simulink library "aeroblk_lib_wf_3dof"  (Simulink 6.0)
settings: Solver=ode45  SolverMode=SingleTasking  StartTime=0.0  StopTime=10.0  RelTol=1e-3
values from neighbouring files (symbols this model uses):
  wf_alphaa = 4.12    [aeroblk_wf_3dof_data.m]
  wf_B3 = 0.06    [aeroblk_wf_3dof_data.m]
  wf_c = 6.5    [aeroblk_wf_3dof_data.m]
  wf_cg = 29    [aeroblk_wf_3dof_data.m]
  wf_cp_e = 112    [aeroblk_wf_3dof_data.m]
  wf_gravity = 32.17    [aeroblk_wf_3dof_data.m]
  wf_H = 16.9    [aeroblk_wf_3dof_data.m]
  wf_incidence = 8    [aeroblk_wf_3dof_data.m]
  wf_Q2 = 1.8    [aeroblk_wf_3dof_data.m]
  wf_Q4 = 2.0    (= 2)    [aeroblk_wf_3dof_data.m]
  wf_sref = 510    [aeroblk_wf_3dof_data.m]
  wf_w2e = 9.7    [aeroblk_wf_3dof_data.m]
  wf_weight = 750    [aeroblk_wf_3dof_data.m]
  wf_z1 = 15    [aeroblk_wf_3dof_data.m]
  wf_z2 = 23    [aeroblk_wf_3dof_data.m]
  wf_z3 = 13    [aeroblk_wf_3dof_data.m]
libraries: simulink x23, aerolibconvert x10, aerolibasang x2, aerolib3dof2 x1, aerolibutil x1, aerolibtransform2 x1, aerolibatmos2 x1, aerolibwind2 x1, aerolibgravity2 x1
settings Model: Creator=The MathWorks Inc.  LastModifiedBy=batserve  ExtModeAutoUpdateStatusClock=off
settings OptimizationCC: BooleanDataType=off
settings DebuggingCC: CheckExecutionContextPreStartOutputMsg=on  CheckExecutionContextRuntimeOutputMsg=on  SolverPrmCheckMsg=none
settings HardwareCC: TargetUnknown=on

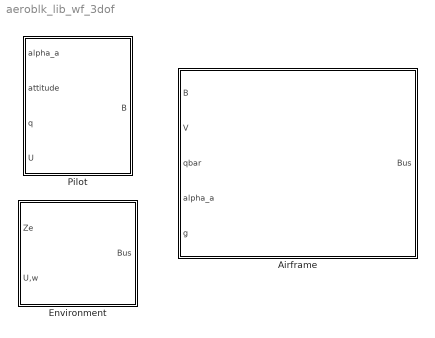
== system aeroblk_lib_wf_3dof ==
  Airframe : Subsystem  PropExecContextAcrossSSBoundary=on
      mask Display: image(imread('aeroblk_wf.jpg'))
  Environment : Subsystem  PropExecContextAcrossSSBoundary=on
      mask Display: image(imread('aeroblk_wf_atmos.jpg'))
  Pilot : Subsystem  PropExecContextAcrossSSBoundary=on
      mask Display: image(imread('aeroblk_orville.jpg'))

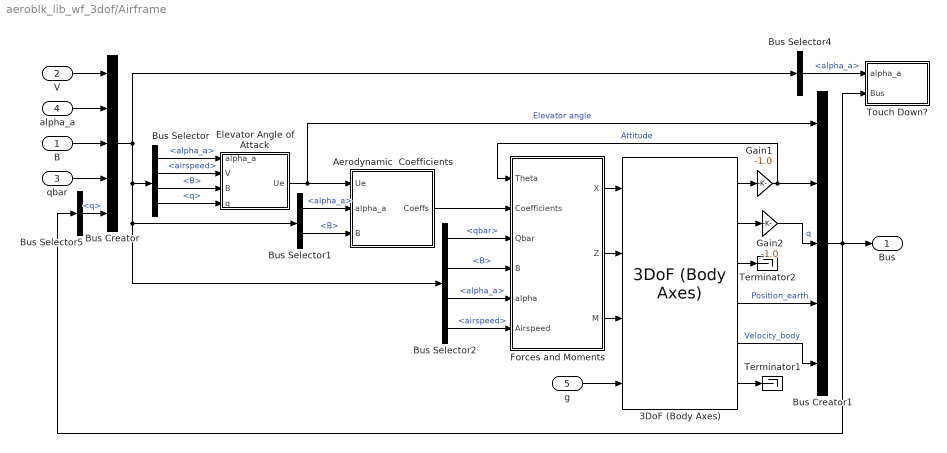
== system aeroblk_lib_wf_3dof/Airframe ==
  "B " : Inport  Port=1  LatchInput=off
  V : Inport  Port=2  LatchInput=off
  qbar : Inport  Port=3  LatchInput=off
  alpha_a : Inport  Port=4  LatchInput=off
  g : Inport  Port=5  LatchInput=off
  3DoF (Body Axes) : aerolib3dof2/3DoF (Body Axes)  units=English (Velocity in ft/s)  mtype=Fixed  v_ini=47.26  theta_ini=-(wf_alphaa-wf_incidence)*pi/180  alpha_ini=wf_alphaa*pi/180  q_ini=wf_q  pos_ini=[0 -0.1]  mass=wf_weight/wf_gravity  mass_e=0.5  mass_f=3.0  Iyy=wf_inertia  Iyy_e=0.5  Iyy_f=3.0  g_in=External  g=wf_gravity
  Aerodynamic  Coefficients : Subsystem  PropExecContextAcrossSSBoundary=on
  Bus Creator : BusCreator  DialogController=Simulink.DDGSource_Bus  Inputs=5
  Bus Creator1 : BusCreator  DialogController=Simulink.DDGSource_Bus  Inputs=5
  Bus Selector : BusSelector  DialogController=Simulink.DDGSource_Bus  OutputSignals=alpha_a,airspeed,B,q
  Bus Selector1 : BusSelector  DialogController=Simulink.DDGSource_Bus  OutputSignals=alpha_a,B
  Bus Selector2 : BusSelector  DialogController=Simulink.DDGSource_Bus  OutputSignals=qbar,B,alpha_a,airspeed
  Bus Selector4 : BusSelector  DialogController=Simulink.DDGSource_Bus  OutputSignals=alpha_a
  Bus Selector5 : BusSelector  DialogController=Simulink.DDGSource_Bus  OutputSignals=q
  "Elevator Angle of Attack " : Subsystem  PropExecContextAcrossSSBoundary=on
  Forces and Moments : Subsystem  PropExecContextAcrossSSBoundary=on
      mask Display:
      | port_label('input',1,'\theta','texmode','on');
      | port_label('input',2,'Coeffs','texmode','on');
      | port_label('input',3,'q_{bar}','texmode','on');
      | port_label('input',4,'B','texmode','on');
      | port_label('input',5,'\alpha','texmode','on');
      | port_label('input',6,'Airspeed','texmode','on');
      | port_label('output',1,'F_x','texmode','on');
      | port_label('output',2,'F_z','texmode','on');
      | port_label('output',3,'M_y','texmode','on');
  Gain1 : Gain  Gain=-1.0  SaturateOnIntegerOverflow=on
  Gain2 : Gain  Gain=-1.0  SaturateOnIntegerOverflow=on
  Terminator1 : Terminator
  Terminator2 : Terminator
  Touch Down? : Subsystem  PropExecContextAcrossSSBoundary=on
  Bus : Outport
  wires:
  Bus Selector5/1 -> Bus Creator/5  "<q>"
  Bus Creator1/1 -> Touch Down?/2(Bus), Bus Selector5/1, Bus/1
  Bus Selector2/1 -> Forces and Moments/3(Qbar)  "<qbar>"
  qbar/1 -> Bus Creator/4
  g/1 -> 3DoF (Body Axes)/4
  3DoF (Body Axes)/3 -> Terminator2/1
  3DoF (Body Axes)/6 -> Terminator1/1
  Gain2/1 -> Bus Creator1/3  "q"
  Gain1/1 -> Forces and Moments/1(Theta), Bus Creator1/2  "Attitude"
  Bus Selector/4 -> "Elevator Angle of Attack "/4(q)  "<q>"
  "Elevator Angle of Attack "/1(Ue) -> Bus Creator1/1, Aerodynamic  Coefficients/1(Ue)  "Elevator angle"
  Bus Selector2/3 -> Forces and Moments/5(alpha)  "<alpha_a>"
  Bus Selector2/2 -> Forces and Moments/4(B)  "<B>"
  Bus Selector1/2 -> Aerodynamic  Coefficients/3(B)  "<B>"
  Bus Selector1/1 -> Aerodynamic  Coefficients/2(alpha_a)  "<alpha_a>"
  Bus Selector/3 -> "Elevator Angle of Attack "/3(B)  "<B>"
  Bus Selector/2 -> "Elevator Angle of Attack "/2(V)  "<airspeed>"
  Bus Selector/1 -> "Elevator Angle of Attack "/1(alpha_a)  "<alpha_a>"
  Bus Creator/1 -> Bus Selector4/1, Bus Selector2/1, Bus Selector1/1, Bus Selector/1
  "B "/1 -> Bus Creator/3
  Bus Selector2/4 -> Forces and Moments/6(Airspeed)  "<airspeed>"
  Bus Selector4/1 -> Touch Down?/1(alpha_a)  "<alpha_a>"
  V/1 -> Bus Creator/1
  3DoF (Body Axes)/5 -> Bus Creator1/5  "Velocity_body"
  3DoF (Body Axes)/4 -> Bus Creator1/4  "Position_earth"
  3DoF (Body Axes)/2 -> Gain2/1
  alpha_a/1 -> Bus Creator/2
  3DoF (Body Axes)/1 -> Gain1/1
  Aerodynamic  Coefficients/1(Coeffs) -> Forces and Moments/2(Coefficients)
  Forces and Moments/1(X) -> 3DoF (Body Axes)/1
  Forces and Moments/2(Z) -> 3DoF (Body Axes)/2
  Forces and Moments/3(M) -> 3DoF (Body Axes)/3

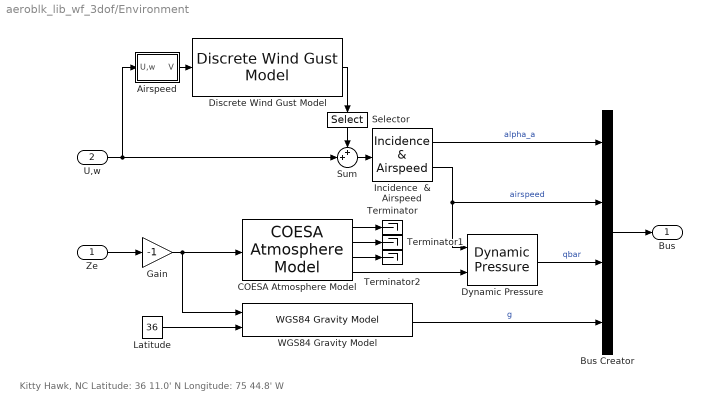
== system aeroblk_lib_wf_3dof/Environment ==
  note: Kitty Hawk, NC
      | Latitude: 36 11.0' N
      | Longitude: 75 44.8' W
  Ze : Inport  Port=1  LatchInput=off
  U,w : Inport  Port=2  LatchInput=off
  Airspeed : Subsystem  PropExecContextAcrossSSBoundary=on
  Bus Creator : BusCreator  DialogController=Simulink.DDGSource_Bus
  COESA Atmosphere Model : aerolibatmos2/COESA Atmosphere Model  units=English (Velocity in ft/s)  spec=1976 COESA-extended U.S. Standard Atmosphere  model=Profile  profile_var=High temperature  profile_percent=1%  profile_alt=5 km (16404 ft)  envelope_var=High temperature  envelope_percent=1%  action=None
  Discrete Wind Gust Model : aerolibwind2/Discrete Wind Gust Model  units=English (Velocity in ft/s)  Gx=off  Gy=off  Gz=off  t_0=0.5  d_m=[120 120 80]  v_m=[3.5 0.0 3.0]
  Dynamic Pressure : aerolibasang/Dynamic Pressure
  Gain : Gain  Gain=-1  SaturateOnIntegerOverflow=on
  Incidence  & Airspeed : aerolibasang/Incidence  & Airspeed
  Latitude : Constant  Value=36
  Selector : Selector  Orientation=down  Elements=[1 3]  InputPortWidth=3
  Sum : Sum  Inputs=++|  SaturateOnIntegerOverflow=on
  Terminator : Terminator
  Terminator1 : Terminator
  Terminator2 : Terminator
  WGS84 Gravity Model : aerolibgravity2/WGS84 Gravity Model  model=WGS84 Taylor Series  units=English  no_atmos=on  precessing=on  month=February  day=1  year=2000  no_centrifugal=on  action=None
  Bus : Outport
  wires:
  Sum/1 -> Incidence  & Airspeed/1
  Bus Creator/1 -> Bus/1
  Latitude/1 -> WGS84 Gravity Model/2
  WGS84 Gravity Model/1 -> Bus Creator/4  "g"
  Gain/1 -> WGS84 Gravity Model/1, COESA Atmosphere Model/1
  Discrete Wind Gust Model/1 -> Selector/1
  U,w/1 -> Sum/2, Airspeed/1(U,w)
  Incidence  & Airspeed/1 -> Bus Creator/1  "alpha_a"
  Incidence  & Airspeed/2 -> Bus Creator/2, Dynamic Pressure/1  "airspeed"
  Dynamic Pressure/1 -> Bus Creator/3  "qbar"
  Ze/1 -> Gain/1
  COESA Atmosphere Model/1 -> Terminator/1
  COESA Atmosphere Model/3 -> Terminator2/1
  COESA Atmosphere Model/2 -> Terminator1/1
  COESA Atmosphere Model/4 -> Dynamic Pressure/2
  Airspeed/1(V) -> Discrete Wind Gust Model/1
  Selector/1 -> Sum/1

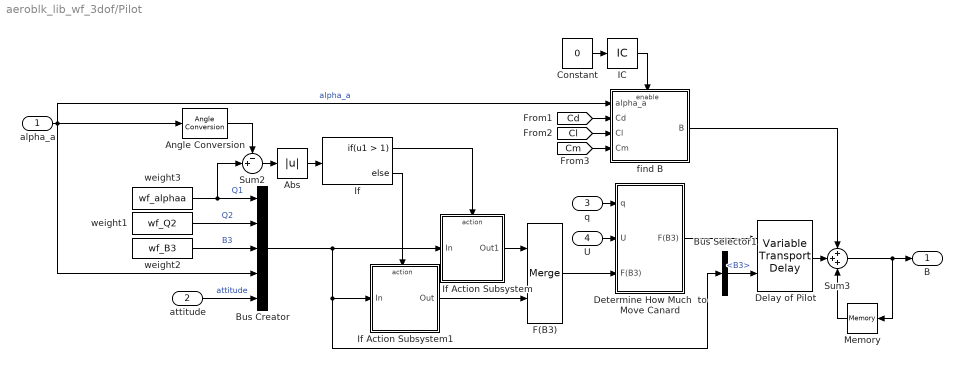
== system aeroblk_lib_wf_3dof/Pilot ==
  alpha_a : Inport  Port=1  LatchInput=off
  attitude : Inport  Port=2  LatchInput=off
  q : Inport  Port=3  LatchInput=off
  U : Inport  Port=4  LatchInput=off
  Abs : Abs  SaturateOnIntegerOverflow=on
  Angle Conversion : aerolibconvert/Angle Conversion  IU=rad  OU=deg
  Bus Creator : BusCreator  DialogController=Simulink.DDGSource_Bus  Inputs=5
  Bus Selector1 : BusSelector  DialogController=Simulink.DDGSource_Bus  OutputSignals=B3
  Constant : Constant  Value=0
  Delay of Pilot : VariableTransportDelay  MaximumDelay=0.08  MaximumPoints=8000
  Determine How Much  to Move Canard : Subsystem  PropExecContextAcrossSSBoundary=on
  F(B3) : Merge
  IC : InitialCondition
  If : If  IfExpression=u1 > 1
  If Action Subsystem : Subsystem  TreatAsAtomicUnit=on  PropExecContextAcrossSSBoundary=on
  If Action Subsystem1 : Subsystem  TreatAsAtomicUnit=on  PropExecContextAcrossSSBoundary=on
  Memory : Memory  Orientation=left  InheritSampleTime=on
  Sum2 : Sum  Inputs=-+|  SaturateOnIntegerOverflow=on
  Sum3 : Sum  Inputs=+++  SaturateOnIntegerOverflow=on
  find B : Subsystem  PropExecContextAcrossSSBoundary=on
  weight1 : Constant  Value=wf_Q2
  weight2 : Constant  Value=wf_B3
  weight3 : Constant  Value=wf_alphaa
  B : Outport
  wires:
  Memory/1 -> Sum3/3
  Constant/1 -> IC/1
  Determine How Much  to Move Canard/1("F(B3) ") -> Delay of Pilot/1
  Bus Selector1/1 -> Delay of Pilot/2  "<B3>"
  weight2/1 -> Bus Creator/3  "B3"
  Delay of Pilot/1 -> Sum3/2
  U/1 -> Determine How Much  to Move Canard/2(U)
  q/1 -> Determine How Much  to Move Canard/1(q)
  F(B3)/1 -> Determine How Much  to Move Canard/3(F(B3))
  [Cm] -> find B/4(Cm)
  [Cl] -> find B/3(Cl)
  IC/1 -> find B/Enable
  [Cd] -> find B/2(Cd)
  find B/1(B) -> Sum3/1
  Sum3/1 -> Memory/1, B/1
  If Action Subsystem1/1(Out) -> F(B3)/2
  If Action Subsystem/1(Out1) -> F(B3)/1
  attitude/1 -> Bus Creator/5  "attitude"
  Bus Creator/1 -> Bus Selector1/1, If Action Subsystem1/1(In), If Action Subsystem/1(In)
  If/2 -> If Action Subsystem1/Action
  weight1/1 -> Bus Creator/2  "Q2"
  If/1 -> If Action Subsystem/Action
  Abs/1 -> If/1
  Sum2/1 -> Abs/1
  Angle Conversion/1 -> Sum2/1
  weight3/1 -> Bus Creator/1, Sum2/2  "Q1"
  alpha_a/1 -> Bus Creator/4, find B/1(alpha_a), Angle Conversion/1  "alpha_a"

== system aeroblk_lib_wf_3dof/Airframe/Aerodynamic  Coefficients ==
  Ue : Inport  Port=1  LatchInput=off
  alpha_a : Inport  Port=2  LatchInput=off
  B : Inport  Port=3  LatchInput=off
  Angle Conversion : aerolibconvert/Angle Conversion  IU=rad  OU=deg
  Bus Creator : BusCreator  DialogController=Simulink.DDGSource_Bus  Inputs=5
  Bus Selector : BusSelector  DialogController=Simulink.DDGSource_Bus  OutputSignals=Cd_wind,Cl_wind,Cm
  Elevator Aerodynamics : Subsystem  PropExecContextAcrossSSBoundary=on
  Wing Aerodynamics : Subsystem  PropExecContextAcrossSSBoundary=on
  Coeffs : Outport
  tag scope: Cd=global, Cl=global, Cm=global
  wires:
  Bus Selector/3 -> [Cm]  "<Cm>"
  Bus Selector/2 -> [Cl]  "<Cl_wind>"
  Bus Selector/1 -> [Cd]  "<Cd_wind>"
  Angle Conversion/1 -> Wing Aerodynamics/1(alpha_a)
  B/1 -> Elevator Aerodynamics/2(B)
  Bus Creator/1 -> Bus Selector/1, Coeffs/1
  Elevator Aerodynamics/2("Cd ") -> Bus Creator/5  "Cd_hs"
  Ue/1 -> Elevator Aerodynamics/1(Ue)
  Elevator Aerodynamics/1(Cl) -> Bus Creator/4  "Cl_hs"
  Wing Aerodynamics/3("Cm ") -> Bus Creator/3  "Cm"
  Wing Aerodynamics/2("Cd ") -> Bus Creator/2  "Cd_wind"
  Wing Aerodynamics/1("Cl ") -> Bus Creator/1  "Cl_wind"
  alpha_a/1 -> Angle Conversion/1

== system aeroblk_lib_wf_3dof/Airframe/Elevator Angle of Attack  ==
  alpha_a : Inport  Port=1  LatchInput=off
  V : Inport  Port=2  LatchInput=off
  B : Inport  Port=3  LatchInput=off
  q : Inport  Port=4  LatchInput=off
  Angle Conversion : aerolibconvert/Angle Conversion  IU=rad  OU=deg
  Calculate Effective  Elevator Angle : Subsystem  PropExecContextAcrossSSBoundary=on
  PreLook-Up Index Search : simulink/Look-Up Tables/PreLook-Up Index Search  bpData=wf_alpha  searchMode=Binary Search  cacheBpFlag=on  outputFlag=off  extrapMode=Linear Extrapolation  rangeErrorMode=None
  Sum1 : Sum  Inputs=+  SaturateOnIntegerOverflow=on
  Sum2 : Sum  Inputs=++|  SaturateOnIntegerOverflow=on
  Ue : Outport
  wires:
  Sum1/1 -> Sum2/2
  q/1 -> Calculate Effective  Elevator Angle/3(q)
  Angle Conversion/1 -> PreLook-Up Index Search/1
  V/1 -> Calculate Effective  Elevator Angle/2(V)
  B/1 -> Calculate Effective  Elevator Angle/1(B)
  alpha_a/1 -> Angle Conversion/1
  PreLook-Up Index Search/1 -> Sum1/1
  Sum2/1 -> Ue/1
  Calculate Effective  Elevator Angle/1(B1) -> Sum2/1

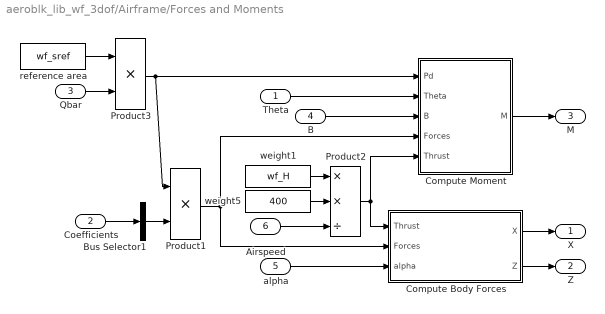
== system aeroblk_lib_wf_3dof/Airframe/Forces and Moments ==
  Theta : Inport  Port=1  LatchInput=off
  Coefficients : Inport  Port=2  LatchInput=off
  Qbar : Inport  Port=3  LatchInput=off
  B : Inport  Port=4  LatchInput=off
  alpha : Inport  Port=5  LatchInput=off
  Airspeed : Inport  Port=6  LatchInput=off
  Bus Selector1 : BusSelector  DialogController=Simulink.DDGSource_Bus  OutputSignals=Cl_wind,Cd_wind,Cm,Cl_hs,Cd_hs  MuxedOutput=on
  Compute Body Forces : Subsystem  PropExecContextAcrossSSBoundary=on
  Compute Moment : Subsystem  PropExecContextAcrossSSBoundary=on
  Product1 : Product  SaturateOnIntegerOverflow=on  InputSameDT=on
  Product2 : Product  Inputs=**/  SaturateOnIntegerOverflow=on  InputSameDT=on
  Product3 : Product  SaturateOnIntegerOverflow=on  InputSameDT=on
  reference area : Constant  Value=wf_sref
  weight1 : Constant  Value=wf_H
  weight5 : Constant  Value=400
  X : Outport
  Z : Outport  Port=2
  M : Outport  Port=3
  wires:
  Airspeed/1 -> Product2/3
  weight1/1 -> Product2/1
  weight5/1 -> Product2/2
  Coefficients/1 -> Bus Selector1/1
  Product3/1 -> Product1/1, Compute Moment/1(Pd)
  Product2/1 -> Compute Moment/5(Thrust), Compute Body Forces/1(Thrust)
  alpha/1 -> Compute Body Forces/3(alpha)
  B/1 -> Compute Moment/3(B)
  Theta/1 -> Compute Moment/2(Theta)
  Compute Moment/1(M) -> M/1
  Product1/1 -> Compute Body Forces/2(Forces), Compute Moment/4(Forces)
  Compute Body Forces/2(Z) -> Z/1
  Compute Body Forces/1(X) -> X/1
  Bus Selector1/1 -> Product1/2
  Qbar/1 -> Product3/2
  reference area/1 -> Product3/1

== system aeroblk_lib_wf_3dof/Airframe/Touch Down? ==
  alpha_a : Inport  Port=1  LatchInput=off
  Bus : Inport  Port=2  LatchInput=off
  Altitude? : simulink/Model Verification/Check Static  Upper Bound  Description=u <= 0  max=0  max_included=on  enabled=on  callback=disp('hitting ground');  stopWhenAssertionFail=off  export=on  icon=graphic
  Bus Selector6 : BusSelector  DialogController=Simulink.DDGSource_Bus  OutputSignals=Elevator angle,Position_earth,Velocity_body,Attitude
  Check Angle of Attack : Subsystem  PropExecContextAcrossSSBoundary=on
  Check Elevator Angle : Subsystem  PropExecContextAcrossSSBoundary=on
  Check Touch Down : Subsystem  TreatAsAtomicUnit=on  PropExecContextAcrossSSBoundary=on
  Selector : Selector  Elements=2  InputPortWidth=2
  Selector1 : Selector  Elements=2  InputPortWidth=2
  Transform  to Earth Axes : Subsystem  PropExecContextAcrossSSBoundary=on
  wires:
  Bus/1 -> Bus Selector6/1
  Selector1/1 -> Altitude?/1
  Altitude?/1 -> Check Touch Down/Trigger
  Bus Selector6/2 -> Selector1/1  "<Position_earth>"
  Selector/1 -> Check Touch Down/1(we)
  Bus Selector6/4 -> Transform  to Earth Axes/2(Theta)  "<Attitude>"
  alpha_a/1 -> Check Angle of Attack/1(alpha_a)
  Bus Selector6/3 -> Transform  to Earth Axes/1(U,w)  "<Velocity_body>"
  Bus Selector6/1 -> Check Elevator Angle/1(Ue)  "<Elevator angle>"
  Transform  to Earth Axes/1(Ue,we) -> Selector/1

== system aeroblk_lib_wf_3dof/Environment/Airspeed ==
  U,w : Inport  Port=1  LatchInput=off
  Airspeed : Math  Operator=sqrt  SaturateOnIntegerOverflow=on
  Dot Product : simulink/Math Operations/Dot Product
  V : Outport
  wires:
  Dot Product/1 -> Airspeed/1
  U,w/1 -> Dot Product/1, Dot Product/2
  Airspeed/1 -> V/1

== system aeroblk_lib_wf_3dof/Pilot/Determine How Much  to Move Canard ==
  q : Inport  Port=1  LatchInput=off
  U : Inport  Port=2  LatchInput=off
  F(B3) : Inport  Port=3  LatchInput=off
  Abs1 : Abs  SaturateOnIntegerOverflow=on
  Don't command a  stall or negative lift situation : Subsystem  PropExecContextAcrossSSBoundary=on
  Gain1 : Gain  Gain=0.002  SaturateOnIntegerOverflow=on
  Product : Product  SaturateOnIntegerOverflow=on
  Relational Operator : RelationalOperator  Operator=<  LogicOutDataTypeMode=Specify via dialog  LogicDataType=float('double')
  Sum1 : Sum  Inputs=-+-  SaturateOnIntegerOverflow=on
  Switch : Switch  Threshold=0.5  SaturateOnIntegerOverflow=on
  Switch2 : Switch  Criteria=u2 > Threshold  Threshold=0.5  SaturateOnIntegerOverflow=on
  weight2 : Constant  Value=0.02
  weight3 : Constant  Value=wf_Q4
  weight5 : Constant  Value=0
  "F(B3) " : Outport
  wires:
  Switch2/1 -> "F(B3) "/1
  weight5/1 -> Switch2/1
  Don't command a  stall or negative lift situation/1(logic) -> Switch2/2
  U/1 -> Don't command a  stall or negative lift situation/1(U)
  Switch/1 -> Switch2/3, Don't command a  stall or negative lift situation/2(F(B3))
  [P] -> Gain1/1
  Gain1/1 -> Sum1/3
  weight3/1 -> Product/2
  Product/1 -> Sum1/1
  Sum1/1 -> Switch/3
  Relational Operator/1 -> Switch/2
  weight2/1 -> Relational Operator/2
  Abs1/1 -> Relational Operator/1
  q/1 -> Product/1, Abs1/1
  F(B3)/1 -> Sum1/2, Switch/1

== system aeroblk_lib_wf_3dof/Pilot/If Action Subsystem ==
  In : Inport  Port=1  LatchInput=off
  Action Port : ActionPort
  Angle Conversion : aerolibconvert/Angle Conversion  IU=deg  OU=rad
  Bus Selector : BusSelector  DialogController=Simulink.DDGSource_Bus  OutputSignals=Q1,alpha_a,Q2
  Product : Product  Inputs=3  SaturateOnIntegerOverflow=on
  Sum2 : Sum  Inputs=+-|  SaturateOnIntegerOverflow=on
  weight1 : Constant  Value=1.5
  Out1 : Outport
  wires:
  Product/1 -> Out1/1
  weight1/1 -> Product/3
  Bus Selector/3 -> Product/2  "<Q2>"
  Sum2/1 -> Product/1
  Angle Conversion/1 -> Sum2/1
  Bus Selector/2 -> Sum2/2  "<alpha_a>"
  Bus Selector/1 -> Angle Conversion/1  "<Q1>"
  In/1 -> Bus Selector/1

== system aeroblk_lib_wf_3dof/Pilot/If Action Subsystem1 ==
  In : Inport  Port=1  LatchInput=off
  Action Port : ActionPort
  Angle Conversion1 : aerolibconvert/Angle Conversion  IU=deg  OU=rad
  Angle Conversion3 : aerolibconvert/Angle Conversion  IU=deg  OU=rad
  Bus Selector1 : BusSelector  DialogController=Simulink.DDGSource_Bus  OutputSignals=Q1,alpha_a,attitude,Q2
  Gain : Gain  Gain=0.5  SaturateOnIntegerOverflow=on
  Product1 : Product  Inputs=3  SaturateOnIntegerOverflow=on
  Sum1 : Sum  Inputs=---  SaturateOnIntegerOverflow=on
  Sum3 : Sum  Inputs=++|  SaturateOnIntegerOverflow=on
  weight2 : Constant  Value=1.5
  weight3 : Constant  Value=wf_incidence
  Out : Outport
  wires:
  Angle Conversion3/1 -> Sum1/3
  Gain/1 -> Sum3/2
  weight3/1 -> Angle Conversion3/1
  Bus Selector1/3 -> Sum1/2  "<attitude>"
  Sum1/1 -> Gain/1
  Product1/1 -> Out/1
  weight2/1 -> Product1/3
  Bus Selector1/4 -> Product1/2  "<Q2>"
  Sum3/1 -> Product1/1
  Angle Conversion1/1 -> Sum3/1
  Bus Selector1/2 -> Sum1/1  "<alpha_a>"
  Bus Selector1/1 -> Angle Conversion1/1  "<Q1>"
  In/1 -> Bus Selector1/1

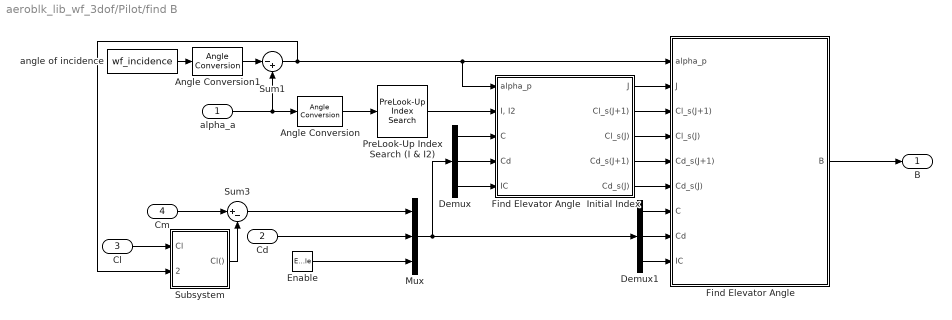
== system aeroblk_lib_wf_3dof/Pilot/find B ==
  alpha_a : Inport  Port=1  LatchInput=off
  Cd : Inport  Port=2  LatchInput=off
  Cl : Inport  Port=3  LatchInput=off
  Cm : Inport  Port=4  LatchInput=off
  Enable : EnablePort  ShowOutputPort=on
  Angle Conversion : aerolibconvert/Angle Conversion  IU=rad  OU=deg
  Angle Conversion1 : aerolibconvert/Angle Conversion  IU=deg  OU=rad
  Demux : Demux  Outputs=3
  Demux1 : Demux  Outputs=3
  Find Elevator Angle : Subsystem  TreatAsAtomicUnit=on  PropExecContextAcrossSSBoundary=on
  Find Elevator Angle  Initial Index : Subsystem  TreatAsAtomicUnit=on  PropExecContextAcrossSSBoundary=on
  Mux : Mux  Inputs=3
  PreLook-Up Index Search (I & I2) : simulink/Look-Up Tables/PreLook-Up Index Search  bpData=wf_alpha  searchMode=Binary Search  cacheBpFlag=on  outputFlag=off  extrapMode=Clip to Range  rangeErrorMode=None
  Subsystem : Subsystem  PropExecContextAcrossSSBoundary=on
  Sum1 : Sum  Inputs=|-+  SaturateOnIntegerOverflow=on
  Sum3 : Sum  Inputs=|+-  SaturateOnIntegerOverflow=on  InputSameDT=on
  angle of incidence : Constant  Value=wf_incidence
  B : Outport  OutputWhenDisabled=reset  InitialOutput=[0]
  wires:
  Subsystem/1(Cl()) -> Sum3/2
  Cm/1 -> Sum3/1
  Cl/1 -> Subsystem/1(Cl)
  Angle Conversion/1 -> PreLook-Up Index Search (I & I2)/1
  Angle Conversion1/1 -> Sum1/1
  angle of incidence/1 -> Angle Conversion1/1
  Enable/1 -> Mux/3
  Find Elevator Angle/1(B) -> B/1
  Mux/1 -> Demux/1, Demux1/1
  Demux1/2 -> Find Elevator Angle/8(Cd)
  Demux/3 -> Find Elevator Angle  Initial Index/5(IC)
  Demux/2 -> Find Elevator Angle  Initial Index/4(Cd)
  Demux/1 -> Find Elevator Angle  Initial Index/3(C)
  Demux1/3 -> Find Elevator Angle/9(IC)
  Demux1/1 -> Find Elevator Angle/7(C)
  Cd/1 -> Mux/2
  Sum3/1 -> Mux/1
  alpha_a/1 -> Angle Conversion/1, Sum1/2
  Find Elevator Angle  Initial Index/5(Cd_s(J)) -> Find Elevator Angle/6(Cd_s(J))
  Find Elevator Angle  Initial Index/4(Cd_s(J+1)) -> Find Elevator Angle/5(Cd_s(J+1))
  Find Elevator Angle  Initial Index/3(Cl_s(J)) -> Find Elevator Angle/4(Cl_s(J))
  Find Elevator Angle  Initial Index/2(Cl_s(J+1)) -> Find Elevator Angle/3(Cl_s(J+1))
  Find Elevator Angle  Initial Index/1(J) -> Find Elevator Angle/2(J)
  Sum1/1 -> Subsystem/2(alpha_p), Find Elevator Angle  Initial Index/1(alpha_p), Find Elevator Angle/1(alpha_p)
  PreLook-Up Index Search (I & I2)/1 -> Find Elevator Angle  Initial Index/2("I, I2")

== system aeroblk_lib_wf_3dof/Airframe/Aerodynamic  Coefficients/Elevator Aerodynamics ==
  Ue : Inport  Port=1  LatchInput=off
  B : Inport  Port=2  LatchInput=off
  Cd : simulink/Look-Up Tables/Interpolation (n-D) using PreLook-Up  numDimsPopupSelect=1  explicitNumDims=2  table=wf_cd  interpMethod=Linear  extrapMethod=Linear  rangeErrorMode=None
  Cls : simulink/Look-Up Tables/Interpolation (n-D) using PreLook-Up  numDimsPopupSelect=1  explicitNumDims=2  table=wf_cls  interpMethod=Linear  extrapMethod=Linear  rangeErrorMode=None
  Constant : Constant  Value=19
  Demux : Demux  Outputs=2
  Gain : Gain  Gain=0.017  SaturateOnIntegerOverflow=on
  Mux : Mux  Inputs=2
  PreLook-Up Index Search : simulink/Look-Up Tables/PreLook-Up Index Search  bpData=wf_alpha2  searchMode=Evenly Spaced Points  cacheBpFlag=on  outputFlag=off  extrapMode=Linear Extrapolation  rangeErrorMode=None
  Product1 : Product  Inputs=*/  SaturateOnIntegerOverflow=on
  Sum : Sum  Inputs=++|  SaturateOnIntegerOverflow=on
  Sum1 : Sum  Inputs=|+-  SaturateOnIntegerOverflow=on
  wing area to  elevator area ratio : Constant  Value=wf_w2e
  Cl : Outport
  "Cd " : Outport  Port=2
  wires:
  Constant/1 -> Sum1/2
  Sum1/1 -> PreLook-Up Index Search/1
  Ue/1 -> Sum1/1
  B/1 -> Gain/1
  Sum/1 -> Mux/1
  Gain/1 -> Sum/1
  Demux/2 -> "Cd "/1
  Demux/1 -> Cl/1
  Mux/1 -> Product1/1
  Product1/1 -> Demux/1
  PreLook-Up Index Search/1 -> Cd/1, Cls/1
  Cd/1 -> Mux/2
  wing area to  elevator area ratio/1 -> Product1/2
  Cls/1 -> Sum/2

== system aeroblk_lib_wf_3dof/Airframe/Aerodynamic  Coefficients/Wing Aerodynamics ==
  alpha_a : Inport  Port=1  LatchInput=off
  Cd : simulink/Look-Up Tables/Interpolation (n-D) using PreLook-Up  numDimsPopupSelect=1  explicitNumDims=2  table=wf_cd  interpMethod=Linear  extrapMethod=Linear  rangeErrorMode=None
  Cl : simulink/Look-Up Tables/Interpolation (n-D) using PreLook-Up  numDimsPopupSelect=1  explicitNumDims=2  table=wf_cl  interpMethod=Linear  extrapMethod=Linear  rangeErrorMode=None
  Cm : simulink/Look-Up Tables/Interpolation (n-D) using PreLook-Up  numDimsPopupSelect=1  explicitNumDims=2  table=wf_cm  interpMethod=Linear  extrapMethod=Linear  rangeErrorMode=None
  PreLook-Up Index Search : simulink/Look-Up Tables/PreLook-Up Index Search  bpData=wf_alpha  searchMode=Evenly Spaced Points  cacheBpFlag=on  outputFlag=off  extrapMode=Linear Extrapolation  rangeErrorMode=None
  PreLook-Up Index Search1 : simulink/Look-Up Tables/PreLook-Up Index Search  bpData=wf_alpha2  searchMode=Evenly Spaced Points  cacheBpFlag=on  outputFlag=off  extrapMode=Linear Extrapolation  rangeErrorMode=None
  "Cl " : Outport
  "Cd " : Outport  Port=2
  "Cm " : Outport  Port=3
  wires:
  PreLook-Up Index Search1/1 -> Cd/1
  Cm/1 -> "Cm "/1
  Cd/1 -> "Cd "/1
  Cl/1 -> "Cl "/1
  alpha_a/1 -> PreLook-Up Index Search1/1, PreLook-Up Index Search/1
  PreLook-Up Index Search/1 -> Cm/1, Cl/1

== system aeroblk_lib_wf_3dof/Airframe/Elevator Angle of Attack /Calculate Effective  Elevator Angle ==
  B : Inport  Port=1  LatchInput=off
  V : Inport  Port=2  LatchInput=off
  q : Inport  Port=3  LatchInput=off
  Angle Conversion : aerolibconvert/Angle Conversion  IU=rad  OU=deg
  Product : Product  Inputs=3  SaturateOnIntegerOverflow=on
  Product1 : Product  SaturateOnIntegerOverflow=on
  Sum : Sum  Inputs=|+-  SaturateOnIntegerOverflow=on
  Sum1 : Sum  Inputs=++|  SaturateOnIntegerOverflow=on
  Trigonometric Function : Trigonometry  Operator=atan2
  weight2 : Constant  Value=100
  weight3 : Constant  Value=wf_c
  weight4 : Constant  Value=wf_cp_e
  weight5 : Constant  Value=wf_cg
  B1 : Outport
  wires:
  Product1/1 -> Trigonometric Function/2
  weight5/1 -> Sum1/1
  weight4/1 -> Sum1/2
  Sum1/1 -> Product/1
  weight3/1 -> Product/2
  weight2/1 -> Product1/1
  q/1 -> Product/3
  V/1 -> Product1/2
  Product/1 -> Trigonometric Function/1
  Trigonometric Function/1 -> Angle Conversion/1
  Angle Conversion/1 -> Sum/2
  Sum/1 -> B1/1
  B/1 -> Sum/1

== system aeroblk_lib_wf_3dof/Airframe/Forces and Moments/Compute Body Forces ==
  Thrust : Inport  Orientation=down  Port=1  LatchInput=off
  Forces : Inport  Port=2  LatchInput=off
  alpha : Inport  Port=3  LatchInput=off
  Convert to body : Subsystem  PropExecContextAcrossSSBoundary=on
  Demux : Demux  Outputs=[2,2]
  Selector : Selector  Elements=[2 5 1 4]  InputPortWidth=5
  Sum3 : Sum  Inputs=1  SaturateOnIntegerOverflow=on  InputSameDT=on
  Sum4 : Sum  Inputs=1  SaturateOnIntegerOverflow=on  InputSameDT=on
  Sum8 : Sum  Inputs=+-|  SaturateOnIntegerOverflow=on  InputSameDT=on
  X : Outport
  Z : Outport  Port=2
  wires:
  Sum8/1 -> Convert to body/1(x-stab force)
  Thrust/1 -> Sum8/1
  Convert to body/2(Z) -> Z/1
  Convert to body/1(X) -> X/1
  Forces/1 -> Selector/1
  Selector/1 -> Demux/1
  alpha/1 -> Convert to body/3(alpha)
  Sum4/1 -> Convert to body/2(lift)  "drag"
  Sum3/1 -> Sum8/2
  Demux/1 -> Sum3/1
  Demux/2 -> Sum4/1

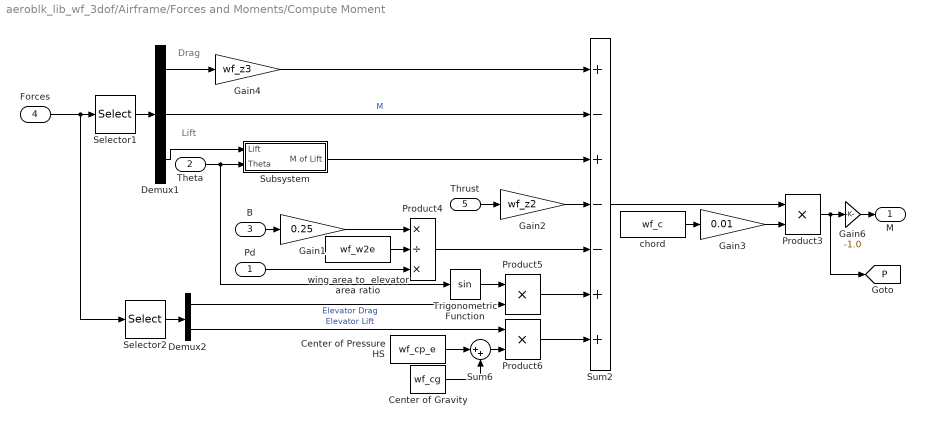
== system aeroblk_lib_wf_3dof/Airframe/Forces and Moments/Compute Moment ==
  note: Lift
  note: Drag
  Pd : Inport  Port=1  LatchInput=off
  Theta : Inport  Port=2  LatchInput=off
  B : Inport  Port=3  LatchInput=off
  Forces : Inport  Port=4  LatchInput=off
  Thrust : Inport  Port=5  LatchInput=off
  Center of Gravity : Constant  Value=wf_cg
  Center of Pressure HS : Constant  Value=wf_cp_e
  Demux1 : Demux  Outputs=3
  Demux2 : Demux  Outputs=2
  Gain1 : Gain  Gain=0.25  SaturateOnIntegerOverflow=on
  Gain2 : Gain  Gain=wf_z2  SaturateOnIntegerOverflow=on
  Gain3 : Gain  Gain=0.01  SaturateOnIntegerOverflow=on
  Gain4 : Gain  Gain=wf_z3  SaturateOnIntegerOverflow=on
  Gain6 : Gain  Gain=-1.0  SaturateOnIntegerOverflow=on
  Product3 : Product  SaturateOnIntegerOverflow=on  InputSameDT=on
  Product4 : Product  Inputs=*/*  SaturateOnIntegerOverflow=on  InputSameDT=on
  Product5 : Product  SaturateOnIntegerOverflow=on  InputSameDT=on
  Product6 : Product  SaturateOnIntegerOverflow=on  InputSameDT=on
  Selector1 : Selector  Elements=[2 3 1]  InputPortWidth=5
  Selector2 : Selector  Elements=[5 4]  InputPortWidth=5
  Subsystem : Subsystem  PropExecContextAcrossSSBoundary=on
  Sum2 : Sum  Inputs=+-+--++  SaturateOnIntegerOverflow=on  InputSameDT=on
  Sum6 : Sum  Inputs=|++  SaturateOnIntegerOverflow=on  InputSameDT=on
  Trigonometric Function : Trigonometry
  chord : Constant  Value=wf_c
  wing area to  elevator area ratio : Constant  Value=wf_w2e
  M : Outport
  tag scope: P=global
  wires:
  Gain2/1 -> Sum2/4
  Gain6/1 -> M/1
  Pd/1 -> Product4/3
  Gain4/1 -> Sum2/1
  Demux2/1 -> Product5/2  "Elevator Drag"
  Demux2/2 -> Product6/1  "Elevator Lift"
  Subsystem/1(M of Lift) -> Sum2/3
  Demux1/2 -> Sum2/2  "M"
  Product3/1 -> [P], Gain6/1
  Thrust/1 -> Gain2/1
  Forces/1 -> Selector2/1, Selector1/1
  Center of Pressure HS/1 -> Sum6/1
  Sum6/1 -> Product6/2
  Center of Gravity/1 -> Sum6/2
  Product6/1 -> Sum2/7
  Product5/1 -> Sum2/6
  Trigonometric Function/1 -> Product5/1
  Selector2/1 -> Demux2/1
  Selector1/1 -> Demux1/1
  Sum2/1 -> Product3/1
  Gain3/1 -> Product3/2
  Theta/1 -> Subsystem/2(Theta), Trigonometric Function/1
  Product4/1 -> Sum2/5
  wing area to  elevator area ratio/1 -> Product4/2
  Gain1/1 -> Product4/1
  B/1 -> Gain1/1
  Demux1/3 -> Subsystem/1(Lift)
  Demux1/1 -> Gain4/1
  chord/1 -> Gain3/1

== system aeroblk_lib_wf_3dof/Airframe/Touch Down?/Check Angle of Attack ==
  alpha_a : Inport  Port=1  LatchInput=off
  Angle Conversion : aerolibconvert/Angle Conversion  IU=rad  OU=deg
  Excess Negative Lift? : simulink/Model Verification/Check Static  Lower Bound  Description=-7 <= u  min=-7  min_included=on  enabled=on  callback=disp('Excess Negative Lift');  stopWhenAssertionFail=off  export=on  icon=graphic
  Logical Operator : Logic  Operator=OR  AllPortsSameDT=off  OutDataTypeMode=Boolean
  Logical Operator2 : Logic  Operator=NOT  AllPortsSameDT=off  OutDataTypeMode=Boolean
  Logical Operator3 : Logic  Operator=NOT  AllPortsSameDT=off  OutDataTypeMode=Boolean
  Stall? : simulink/Model Verification/Check Static  Upper Bound  Description=u <= 50  max=50  max_included=on  enabled=on  callback=disp('Stall');  stopWhenAssertionFail=off  export=on  icon=graphic
  Stop Simulation : Stop
  wires:
  Angle Conversion/1 -> Stall?/1, Excess Negative Lift?/1
  alpha_a/1 -> Angle Conversion/1
  Stall?/1 -> Logical Operator2/1
  Excess Negative Lift?/1 -> Logical Operator3/1
  Logical Operator/1 -> Stop Simulation/1
  Logical Operator2/1 -> Logical Operator/1
  Logical Operator3/1 -> Logical Operator/2

== system aeroblk_lib_wf_3dof/Airframe/Touch Down?/Check Elevator Angle ==
  Ue : Inport  Port=1  LatchInput=off
  Elevator Stall? : simulink/Model Verification/Check Static  Upper Bound  Description=u <= 110  max=110  max_included=on  enabled=on  callback=disp('Elevator Stall');  stopWhenAssertionFail=off  export=on  icon=graphic
  Excess Negative Elevator? : simulink/Model Verification/Check Static  Lower Bound  Description=2 <= u  min=2  min_included=on  enabled=on  callback=disp('Excess Negative Elevator');  stopWhenAssertionFail=off  export=on  icon=graphic
  Logical Operator : Logic  Operator=OR  AllPortsSameDT=off  OutDataTypeMode=Boolean
  Logical Operator1 : Logic  Operator=NOT  AllPortsSameDT=off  OutDataTypeMode=Boolean
  Logical Operator2 : Logic  Operator=NOT  AllPortsSameDT=off  OutDataTypeMode=Boolean
  Stop Simulation : Stop
  wires:
  Ue/1 -> Excess Negative Elevator?/1, Elevator Stall?/1
  Elevator Stall?/1 -> Logical Operator2/1
  Excess Negative Elevator?/1 -> Logical Operator1/1
  Logical Operator/1 -> Stop Simulation/1
  Logical Operator1/1 -> Logical Operator/2
  Logical Operator2/1 -> Logical Operator/1

== system aeroblk_lib_wf_3dof/Airframe/Touch Down?/Check Touch Down ==
  we : Inport  Port=1  LatchInput=off
  Trigger : TriggerPort  TriggerType=falling
  Crash? : simulink/Model Verification/Check Static  Upper Bound  Description=u < 10  max=10  max_included=off  enabled=on  callback=disp('Crash');  stopWhenAssertionFail=off  export=on  icon=graphic
  Hard Landing? : simulink/Model Verification/Check  Static Gap  Description=u <= 6 || 10 <= u  max=10  max_included=on  min=6  min_included=on  enabled=on  callback=disp('Hard Landing');  stopWhenAssertionFail=off  export=on  icon=graphic
  Land? : simulink/Model Verification/Check Static  Lower Bound  Description=6 < u  min=6  min_included=off  enabled=on  callback=disp('Landing');  stopWhenAssertionFail=off  export=on  icon=graphic
  Logical Operator : Logic  Operator=OR  Inputs=3  AllPortsSameDT=off  OutDataTypeMode=Boolean
  Logical Operator1 : Logic  Operator=NOT  AllPortsSameDT=off  OutDataTypeMode=Boolean
  Logical Operator2 : Logic  Operator=NOT  AllPortsSameDT=off  OutDataTypeMode=Boolean
  Logical Operator3 : Logic  Operator=NOT  AllPortsSameDT=off  OutDataTypeMode=Boolean
  Stop Simulation : Stop
  wires:
  we/1 -> Land?/1, Crash?/1, Hard Landing?/1
  Land?/1 -> Logical Operator2/1
  Logical Operator/1 -> Stop Simulation/1
  Hard Landing?/1 -> Logical Operator3/1
  Crash?/1 -> Logical Operator1/1
  Logical Operator1/1 -> Logical Operator/3
  Logical Operator2/1 -> Logical Operator/1
  Logical Operator3/1 -> Logical Operator/2

== system aeroblk_lib_wf_3dof/Airframe/Touch Down?/Transform  to Earth Axes ==
  U,w : Inport  Port=1  LatchInput=off
  Theta : Inport  Port=2  LatchInput=off
  Constant : Constant  Value=0
  Euler Angles to  Direction Cosine Matrix : aerolibtransform2/Euler Angles to  Direction Cosine Matrix
  Gain1 : Gain  Gain=-1.0  SaturateOnIntegerOverflow=on
  Mux3 : Mux  Inputs=3
  Mux4 : Mux  Inputs=3
  Product : Product  Multiplication=Matrix(*)  SaturateOnIntegerOverflow=on
  Selector : Selector  InputPortWidth=2
  Selector1 : Selector  Elements=[1 3]  InputPortWidth=3
  Selector2 : Selector  Elements=2  InputPortWidth=2
  Transpose : Math  Operator=transpose  SaturateOnIntegerOverflow=on
  Ue,we : Outport
  wires:
  Gain1/1 -> Mux3/2
  Transpose/1 -> Product/1
  Theta/1 -> Gain1/1
  U,w/1 -> Selector/1, Selector2/1
  Mux3/1 -> Euler Angles to  Direction Cosine Matrix/1
  Constant/1 -> Mux3/1, Mux3/3, Mux4/2
  Euler Angles to  Direction Cosine Matrix/1 -> Transpose/1
  Mux4/1 -> Product/2
  Product/1 -> Selector1/1
  Selector1/1 -> Ue,we/1
  Selector/1 -> Mux4/1
  Selector2/1 -> Mux4/3

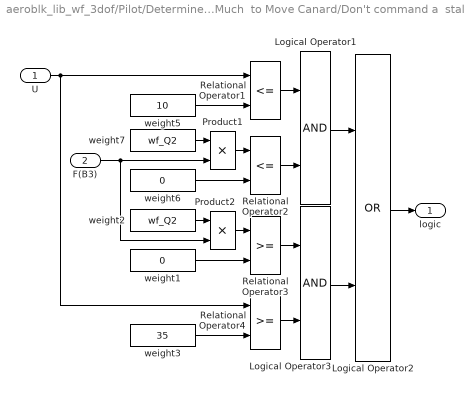
== system aeroblk_lib_wf_3dof/Pilot/Determine How Much  to Move Canard/Don't command a  stall or negative lift situation ==
  U : Inport  Port=1  LatchInput=off
  F(B3) : Inport  Port=2  LatchInput=off
  Logical Operator1 : Logic  AllPortsSameDT=off  OutDataTypeMode=Specify via dialog  LogicDataType=float('double')
  Logical Operator2 : Logic  Operator=OR  AllPortsSameDT=off  OutDataTypeMode=Specify via dialog  LogicDataType=float('double')
  Logical Operator3 : Logic  AllPortsSameDT=off  OutDataTypeMode=Specify via dialog  LogicDataType=float('double')
  Product1 : Product  SaturateOnIntegerOverflow=on
  Product2 : Product  SaturateOnIntegerOverflow=on
  Relational Operator1 : RelationalOperator  Operator=<=
  Relational Operator2 : RelationalOperator  Operator=<=
  Relational Operator3 : RelationalOperator
  Relational Operator4 : RelationalOperator
  weight1 : Constant  Value=0
  weight2 : Constant  Value=wf_Q2
  weight3 : Constant  Value=35
  weight5 : Constant  Value=10
  weight6 : Constant  Value=0
  weight7 : Constant  Value=wf_Q2
  logic : Outport
  wires:
  Logical Operator3/1 -> Logical Operator2/2
  Logical Operator1/1 -> Logical Operator2/1
  weight3/1 -> Relational Operator4/2
  Relational Operator4/1 -> Logical Operator3/2
  Product2/1 -> Relational Operator3/1
  weight2/1 -> Product2/1
  weight1/1 -> Relational Operator3/2
  Relational Operator3/1 -> Logical Operator3/1
  Logical Operator2/1 -> logic/1
  F(B3)/1 -> Product1/2, Product2/2
  weight7/1 -> Product1/1
  Product1/1 -> Relational Operator2/1
  weight6/1 -> Relational Operator2/2
  Relational Operator2/1 -> Logical Operator1/2
  Relational Operator1/1 -> Logical Operator1/1
  weight5/1 -> Relational Operator1/2
  U/1 -> Relational Operator4/1, Relational Operator1/1

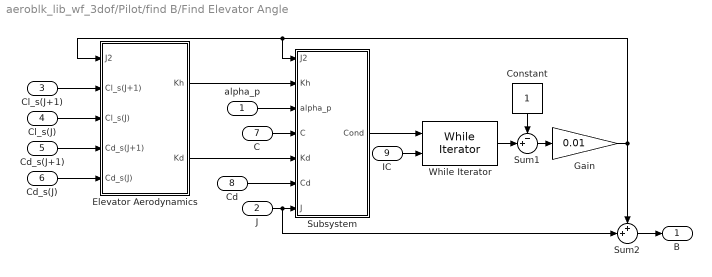
== system aeroblk_lib_wf_3dof/Pilot/find B/Find Elevator Angle ==
  alpha_p : Inport  Port=1  LatchInput=off
  J : Inport  Port=2  LatchInput=off
  Cl_s(J+1) : Inport  Port=3  LatchInput=off
  Cl_s(J) : Inport  Port=4  LatchInput=off
  Cd_s(J+1) : Inport  Port=5  LatchInput=off
  Cd_s(J) : Inport  Port=6  LatchInput=off
  C : Inport  Port=7  LatchInput=off
  Cd : Inport  Port=8  LatchInput=off
  IC : Inport  Port=9  LatchInput=off
  Constant : Constant  Orientation=down
  Elevator Aerodynamics : Subsystem  PropExecContextAcrossSSBoundary=on
  Gain : Gain  Gain=0.01  SaturateOnIntegerOverflow=on
  Subsystem : Subsystem  PropExecContextAcrossSSBoundary=on
  Sum1 : Sum  Inputs=-+|  SaturateOnIntegerOverflow=on
  Sum2 : Sum  Inputs=++|  SaturateOnIntegerOverflow=on
  While Iterator : WhileIterator  MaxIters=100  ShowIterationPort=on  OutputDataType=double
  B : Outport
  wires:
  Cd_s(J)/1 -> Elevator Aerodynamics/5(Cd_s(J))
  Cd_s(J+1)/1 -> Elevator Aerodynamics/4(Cd_s(J+1))
  Cl_s(J)/1 -> Elevator Aerodynamics/3(Cl_s(J))
  Cl_s(J+1)/1 -> Elevator Aerodynamics/2(Cl_s(J+1))
  Sum2/1 -> B/1
  Constant/1 -> Sum1/1
  Sum1/1 -> Gain/1
  Gain/1 -> Subsystem/1(J2), Elevator Aerodynamics/1(J2), Sum2/1
  J/1 -> Sum2/2, Subsystem/7(J)
  While Iterator/1 -> Sum1/2
  alpha_p/1 -> Subsystem/3(alpha_p)
  Elevator Aerodynamics/2("Kd ") -> Subsystem/5(Kd)
  Elevator Aerodynamics/1(Kh) -> Subsystem/2(Kh)
  Subsystem/1(Cond) -> While Iterator/1
  C/1 -> Subsystem/4(C)
  Cd/1 -> Subsystem/6(Cd)
  IC/1 -> While Iterator/2

== system aeroblk_lib_wf_3dof/Pilot/find B/Find Elevator Angle  Initial Index ==
  alpha_p : Inport  Port=1  LatchInput=off
  "I, I2" : Inport  Port=2  LatchInput=off
  C : Inport  Port=3  LatchInput=off
  Cd : Inport  Port=4  LatchInput=off
  IC : Inport  Port=5  LatchInput=off
  Constant : Constant  Orientation=down
  Demux : Demux  Outputs=2
  Elevator Aerodynamics : Subsystem  PropExecContextAcrossSSBoundary=on
  Subsystem : Subsystem  PropExecContextAcrossSSBoundary=on
  Sum1 : Sum  Inputs=-+|  SaturateOnIntegerOverflow=on
  While Iterator : WhileIterator  MaxIters=-1  ShowIterationPort=on  OutputDataType=double
  J : Outport
  Cl_s(J+1) : Outport  Port=2
  Cl_s(J) : Outport  Port=3
  Cd_s(J+1) : Outport  Port=4
  Cd_s(J) : Outport  Port=5
  wires:
  Elevator Aerodynamics/2(Cl_s(J)) -> Cl_s(J)/1
  Elevator Aerodynamics/3(Cd_s(J)) -> Cd_s(J)/1
  Constant/1 -> Sum1/1
  Sum1/1 -> J/1
  IC/1 -> While Iterator/2
  Cd/1 -> Subsystem/6(Cd)
  C/1 -> Subsystem/5(C)
  Subsystem/1(Cond) -> While Iterator/1
  Elevator Aerodynamics/1(Cl_s(J+1)) -> Cl_s(J+1)/1, Subsystem/2(Cl_s)
  Elevator Aerodynamics/4(Cd_s(J+1)) -> Cd_s(J+1)/1, Subsystem/4(Cd_s)
  alpha_p/1 -> Subsystem/3(alpha_p)
  Demux/1 -> Elevator Aerodynamics/2(I), Subsystem/7(I)
  While Iterator/1 -> Elevator Aerodynamics/1(J+1), Sum1/2, Subsystem/1(J)
  Demux/2 -> Elevator Aerodynamics/3(I2)
  "I, I2"/1 -> Demux/1

== system aeroblk_lib_wf_3dof/Pilot/find B/Subsystem ==
  Cl : Inport  Port=1  LatchInput=off
  alpha_p : Inport  Port=2  LatchInput=off
  Center of Gravity : Constant  Value=wf_cg
  Center of Pressure : Constant  Value=wf_z1
  Product1 : Product  SaturateOnIntegerOverflow=on  InputSameDT=on
  Product5 : Product  SaturateOnIntegerOverflow=on  InputSameDT=on
  Sum2 : Sum  Inputs=-+|  SaturateOnIntegerOverflow=on  InputSameDT=on
  Trigonometric Function : Trigonometry
  Cl() : Outport
  wires:
  Cl/1 -> Product1/2
  Product1/1 -> Cl()/1
  Sum2/1 -> Product1/1
  alpha_p/1 -> Trigonometric Function/1
  Trigonometric Function/1 -> Product5/1
  Product5/1 -> Sum2/1
  Center of Gravity/1 -> Sum2/2
  Center of Pressure/1 -> Product5/2

== system aeroblk_lib_wf_3dof/Airframe/Forces and Moments/Compute Body Forces/Convert to body ==
  note: weight is accounted
      | for in 3DoF model
  x-stab force : Inport  Port=1  LatchInput=off
  lift : Inport  Port=2  LatchInput=off
  alpha : Inport  Port=3  LatchInput=off
  Gain1 : Gain  Gain=-1  SaturateOnIntegerOverflow=on
  Mux : Mux  Inputs=2
  Mux1 : Mux  Inputs=2
  Product1 : Product  SaturateOnIntegerOverflow=on  InputSameDT=on
  Product3 : Product  SaturateOnIntegerOverflow=on  InputSameDT=on
  Selector : Selector  Elements=[2 3]  InputPortWidth=4
  Selector1 : Selector  Elements=[1 4]  InputPortWidth=4
  SinCos : aerolibutil/SinCos
  Sum1 : Sum  Inputs=1  SaturateOnIntegerOverflow=on  InputSameDT=on
  Sum3 : Sum  Inputs=1  SaturateOnIntegerOverflow=on  InputSameDT=on
  X : Outport
  Z : Outport  Port=2
  wires:
  Gain1/1 -> Product3/2
  alpha/1 -> SinCos/1
  Sum1/1 -> Z/1
  Sum3/1 -> X/1
  Selector1/1 -> Sum1/1
  Selector/1 -> Sum3/1
  Mux1/1 -> Selector/1, Selector1/1
  Product1/1 -> Mux1/1
  Product3/1 -> Mux1/2
  x-stab force/1 -> Product1/1
  lift/1 -> Gain1/1  "lift"
  Mux/1 -> Product3/1, Product1/2
  SinCos/2 -> Mux/2
  SinCos/1 -> Mux/1

== system aeroblk_lib_wf_3dof/Airframe/Forces and Moments/Compute Moment/Subsystem ==
  Lift : Inport  Port=1  LatchInput=off
  Theta : Inport  Port=2  LatchInput=off
  Center of Gravity : Constant  Value=wf_cg
  Center of Pressure : Constant  Value=wf_z1
  Product1 : Product  SaturateOnIntegerOverflow=on  InputSameDT=on
  Product5 : Product  SaturateOnIntegerOverflow=on  InputSameDT=on
  Sum2 : Sum  Inputs=-+|  SaturateOnIntegerOverflow=on  InputSameDT=on
  Trigonometric Function : Trigonometry
  M of Lift : Outport
  wires:
  Lift/1 -> Product1/2
  Product1/1 -> M of Lift/1
  Sum2/1 -> Product1/1
  Theta/1 -> Trigonometric Function/1
  Trigonometric Function/1 -> Product5/1
  Product5/1 -> Sum2/1
  Center of Gravity/1 -> Sum2/2
  Center of Pressure/1 -> Product5/2

== system aeroblk_lib_wf_3dof/Pilot/find B/Find Elevator Angle/Elevator Aerodynamics ==
  J2 : Inport  Port=1  LatchInput=off
  Cl_s(J+1) : Inport  Port=2  LatchInput=off
  Cl_s(J) : Inport  Port=3  LatchInput=off
  Cd_s(J+1) : Inport  Port=4  LatchInput=off
  Cd_s(J) : Inport  Port=5  LatchInput=off
  Product : Product  SaturateOnIntegerOverflow=on
  Product1 : Product  SaturateOnIntegerOverflow=on
  Sum : Sum  Inputs=|++  SaturateOnIntegerOverflow=on
  Sum1 : Sum  Inputs=|++  SaturateOnIntegerOverflow=on
  Sum2 : Sum  Inputs=|+-  SaturateOnIntegerOverflow=on
  Sum3 : Sum  Inputs=-+|  SaturateOnIntegerOverflow=on
  Kh : Outport
  "Kd " : Outport  Port=2
  wires:
  Cl_s(J)/1 -> Sum3/1, Sum1/1
  Cl_s(J+1)/1 -> Sum3/2
  Sum3/1 -> Product1/1
  Cd_s(J)/1 -> Sum/2, Sum2/2
  Cd_s(J+1)/1 -> Sum2/1
  Sum2/1 -> Product/2
  Product1/1 -> Sum1/2
  J2/1 -> Product1/2, Product/1
  Product/1 -> Sum/1
  Sum/1 -> "Kd "/1
  Sum1/1 -> Kh/1

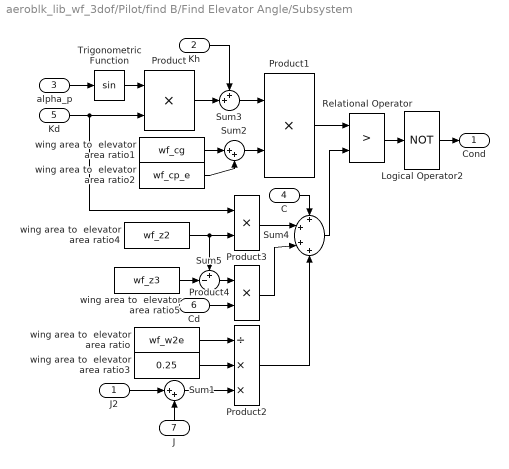
== system aeroblk_lib_wf_3dof/Pilot/find B/Find Elevator Angle/Subsystem ==
  J2 : Inport  Port=1  LatchInput=off
  Kh : Inport  Port=2  LatchInput=off
  alpha_p : Inport  Port=3  LatchInput=off
  C : Inport  Port=4  LatchInput=off
  Kd : Inport  Port=5  LatchInput=off
  Cd : Inport  Port=6  LatchInput=off
  J : Inport  Orientation=up  Port=7  LatchInput=off
  Logical Operator2 : Logic  Operator=NOT  AllPortsSameDT=off
  Product{,1,3..4} (4 alike) : Product  SaturateOnIntegerOverflow=on
  Product2 : Product  Inputs=/**  SaturateOnIntegerOverflow=on
  Relational Operator : RelationalOperator  Operator=>
  Sum1 : Sum  Inputs=|++  SaturateOnIntegerOverflow=on
  Sum2 : Sum  Inputs=|++  SaturateOnIntegerOverflow=on
  Sum3 : Sum  Inputs=++|  SaturateOnIntegerOverflow=on
  Sum4 : Sum  Inputs=++++  SaturateOnIntegerOverflow=on
  Sum5 : Sum  Inputs=+-|  SaturateOnIntegerOverflow=on
  Trigonometric Function : Trigonometry
  wing area to  elevator area ratio : Constant  Value=wf_w2e
  wing area to  elevator area ratio1 : Constant  Value=wf_cg
  wing area to  elevator area ratio2 : Constant  Value=wf_cp_e
  wing area to  elevator area ratio3 : Constant  Value=0.25
  wing area to  elevator area ratio4 : Constant  Value=wf_z2
  wing area to  elevator area ratio5 : Constant  Value=wf_z3
  Cond : Outport
  wires:
  Product4/1 -> Sum4/3
  Logical Operator2/1 -> Cond/1
  wing area to  elevator area ratio2/1 -> Sum2/2
  wing area to  elevator area ratio1/1 -> Sum2/1
  Trigonometric Function/1 -> Product/1
  Product/1 -> Sum3/2
  Sum3/1 -> Product1/1
  Sum2/1 -> Product1/2
  Product1/1 -> Relational Operator/1
  Sum1/1 -> Product2/3
  Relational Operator/1 -> Logical Operator2/1
  J2/1 -> Sum1/1
  J/1 -> Sum1/2
  Kh/1 -> Sum3/1
  alpha_p/1 -> Trigonometric Function/1
  Kd/1 -> Product3/1, Product/2
  Sum4/1 -> Relational Operator/2
  C/1 -> Sum4/1
  Product2/1 -> Sum4/4
  wing area to  elevator area ratio/1 -> Product2/1
  wing area to  elevator area ratio3/1 -> Product2/2
  wing area to  elevator area ratio4/1 -> Product3/2, Sum5/1
  wing area to  elevator area ratio5/1 -> Sum5/2
  Sum5/1 -> Product4/1
  Cd/1 -> Product4/2
  Product3/1 -> Sum4/2

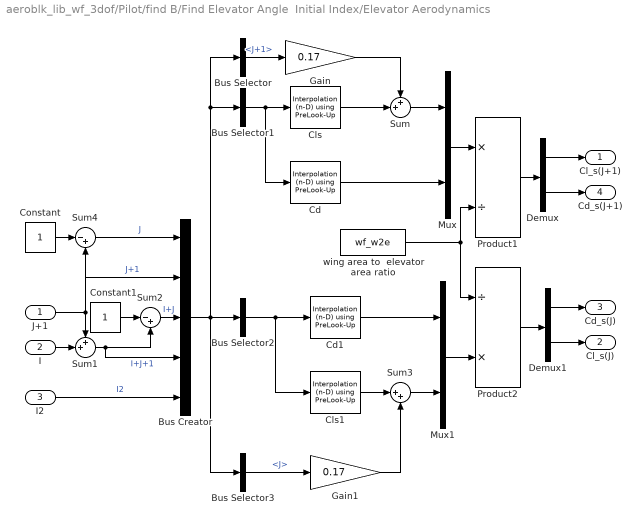
== system aeroblk_lib_wf_3dof/Pilot/find B/Find Elevator Angle  Initial Index/Elevator Aerodynamics ==
  J+1 : Inport  Port=1  LatchInput=off
  I : Inport  Port=2  LatchInput=off
  I2 : Inport  Port=3  LatchInput=off
  Bus Creator : BusCreator  DialogController=Simulink.DDGSource_Bus  Inputs=5
  Bus Selector : BusSelector  DialogController=Simulink.DDGSource_Bus  OutputSignals=J+1
  Bus Selector1 : BusSelector  DialogController=Simulink.DDGSource_Bus  OutputSignals=I+J+1,I2  MuxedOutput=on
  Bus Selector2 : BusSelector  DialogController=Simulink.DDGSource_Bus  OutputSignals=I+J,I2  MuxedOutput=on
  Bus Selector3 : BusSelector  DialogController=Simulink.DDGSource_Bus  OutputSignals=J
  Cd : simulink/Look-Up Tables/Interpolation (n-D) using PreLook-Up  numDimsPopupSelect=1  explicitNumDims=2  table=wf_cd  interpMethod=Linear  extrapMethod=Linear  rangeErrorMode=None
  Cd1 : simulink/Look-Up Tables/Interpolation (n-D) using PreLook-Up  numDimsPopupSelect=1  explicitNumDims=2  table=wf_cd  interpMethod=Linear  extrapMethod=Linear  rangeErrorMode=None
  Cls : simulink/Look-Up Tables/Interpolation (n-D) using PreLook-Up  numDimsPopupSelect=1  explicitNumDims=2  table=wf_cls  interpMethod=Linear  extrapMethod=Linear  rangeErrorMode=None
  Cls1 : simulink/Look-Up Tables/Interpolation (n-D) using PreLook-Up  numDimsPopupSelect=1  explicitNumDims=2  table=wf_cls  interpMethod=Linear  extrapMethod=Linear  rangeErrorMode=None
  Constant : Constant
  Constant1 : Constant
  Demux : Demux  Outputs=2
  Demux1 : Demux  Outputs=2
  Gain : Gain  Gain=0.17  SaturateOnIntegerOverflow=on
  Gain1 : Gain  Gain=0.17  SaturateOnIntegerOverflow=on
  Mux : Mux  Inputs=2
  Mux1 : Mux  Inputs=2
  Product1 : Product  Inputs=*/  SaturateOnIntegerOverflow=on
  Product2 : Product  Inputs=/*  SaturateOnIntegerOverflow=on
  Sum : Sum  Inputs=++|  SaturateOnIntegerOverflow=on
  Sum1 : Sum  Inputs=++|  SaturateOnIntegerOverflow=on
  Sum2 : Sum  Inputs=|-+  SaturateOnIntegerOverflow=on
  Sum3 : Sum  Inputs=|++  SaturateOnIntegerOverflow=on
  Sum4 : Sum  Inputs=|-+  SaturateOnIntegerOverflow=on
  wing area to  elevator area ratio : Constant  Value=wf_w2e
  Cl_s(J+1) : Outport
  Cl_s(J) : Outport  Port=2
  Cd_s(J) : Outport  Port=3
  Cd_s(J+1) : Outport  Port=4
  wires:
  Bus Selector3/1 -> Gain1/1  "<J>"
  Bus Selector2/1 -> Cls1/1, Cd1/1
  Bus Selector/1 -> Gain/1  "<J+1>"
  Bus Creator/1 -> Bus Selector3/1, Bus Selector2/1, Bus Selector1/1, Bus Selector/1
  Sum4/1 -> Bus Creator/1  "J"
  Constant1/1 -> Sum2/1
  Constant/1 -> Sum4/1
  Cls1/1 -> Sum3/1
  Sum3/1 -> Mux1/2
  Gain1/1 -> Sum3/2
  Cd1/1 -> Mux1/1
  Mux1/1 -> Product2/2
  Demux1/2 -> Cl_s(J)/1
  Demux1/1 -> Cd_s(J)/1
  Product2/1 -> Demux1/1
  Sum2/1 -> Bus Creator/3  "I+J"
  Sum1/1 -> Bus Creator/4, Sum2/2  "I+J+1"
  I2/1 -> Bus Creator/5  "I2"
  Bus Selector1/1 -> Cd/1, Cls/1
  I/1 -> Sum1/2
  J+1/1 -> Bus Creator/2, Sum4/2, Sum1/1  "J+1"
  Cls/1 -> Sum/2
  wing area to  elevator area ratio/1 -> Product2/1, Product1/2
  Cd/1 -> Mux/2
  Product1/1 -> Demux/1
  Mux/1 -> Product1/1
  Demux/1 -> Cl_s(J+1)/1
  Demux/2 -> Cd_s(J+1)/1
  Gain/1 -> Sum/1
  Sum/1 -> Mux/1

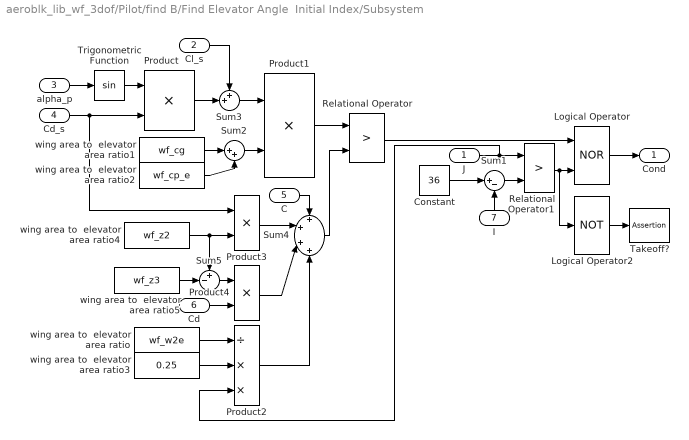
== system aeroblk_lib_wf_3dof/Pilot/find B/Find Elevator Angle  Initial Index/Subsystem ==
  J : Inport  Port=1  LatchInput=off
  Cl_s : Inport  Port=2  LatchInput=off
  alpha_p : Inport  Port=3  LatchInput=off
  Cd_s : Inport  Port=4  LatchInput=off
  C : Inport  Port=5  LatchInput=off
  Cd : Inport  Port=6  LatchInput=off
  I : Inport  Orientation=up  Port=7  LatchInput=off
  Constant : Constant  Value=36
  Logical Operator : Logic  Operator=NOR  AllPortsSameDT=off
  Logical Operator2 : Logic  Operator=NOT  AllPortsSameDT=off
  Product{,1,3..4} (4 alike) : Product  SaturateOnIntegerOverflow=on
  Product2 : Product  Inputs=/**  SaturateOnIntegerOverflow=on
  Relational Operator : RelationalOperator  Operator=>
  Relational Operator1 : RelationalOperator  Operator=>
  Sum1 : Sum  Inputs=|+-  SaturateOnIntegerOverflow=on
  Sum2 : Sum  Inputs=|++  SaturateOnIntegerOverflow=on
  Sum3 : Sum  Inputs=++|  SaturateOnIntegerOverflow=on
  Sum4 : Sum  Inputs=++++  SaturateOnIntegerOverflow=on
  Sum5 : Sum  Inputs=+-|  SaturateOnIntegerOverflow=on
  Takeoff? : Assertion  AssertionFailFcn=disp('No Takeoff');
  Trigonometric Function : Trigonometry
  wing area to  elevator area ratio : Constant  Value=wf_w2e
  wing area to  elevator area ratio1 : Constant  Value=wf_cg
  wing area to  elevator area ratio2 : Constant  Value=wf_cp_e
  wing area to  elevator area ratio3 : Constant  Value=0.25
  wing area to  elevator area ratio4 : Constant  Value=wf_z2
  wing area to  elevator area ratio5 : Constant  Value=wf_z3
  Cond : Outport
  wires:
  Logical Operator2/1 -> Takeoff?/1
  Product3/1 -> Sum4/2
  Product4/1 -> Sum4/3
  Cd/1 -> Product4/2
  Sum5/1 -> Product4/1
  wing area to  elevator area ratio5/1 -> Sum5/2
  wing area to  elevator area ratio4/1 -> Sum5/1, Product3/2
  wing area to  elevator area ratio3/1 -> Product2/2
  wing area to  elevator area ratio/1 -> Product2/1
  Product2/1 -> Sum4/4
  C/1 -> Sum4/1
  Sum4/1 -> Relational Operator/2
  Cd_s/1 -> Product3/1, Product/2
  alpha_p/1 -> Trigonometric Function/1
  Cl_s/1 -> Sum3/1
  Logical Operator/1 -> Cond/1
  I/1 -> Sum1/2
  J/1 -> Product2/3, Relational Operator1/1
  Relational Operator/1 -> Logical Operator/1
  Relational Operator1/1 -> Logical Operator2/1, Logical Operator/2
  Sum1/1 -> Relational Operator1/2
  Product1/1 -> Relational Operator/1
  Sum2/1 -> Product1/2
  Sum3/1 -> Product1/1
  Product/1 -> Sum3/2
  Trigonometric Function/1 -> Product/1
  wing area to  elevator area ratio1/1 -> Sum2/1
  wing area to  elevator area ratio2/1 -> Sum2/2
  Constant/1 -> Sum1/1
